simulink model "VCU_CS75_9_30"  (R2014a)
settings: Solver=FixedStepDiscrete  StartTime=0.0  StopTime=25  FixedStep=0.0005  RelTol=1e-3
undefined symbols (not defined in the file or in its folder): APAStatus_2D4, ecucoder_acal, I_SW01_L, LDW, ST_comd, TX2D4
libraries: simulink x881, ec5744lib x37
(part 24 of 30)

== system VCU_CS75_9_30/长安CS75底盘程序，20ms一次/BSW_Input/CAN1_Rx/BCM_3DF/ReceiveMessages/Subsystem/BCM_3DF1 ==
  input : Inport
  BCM_AmbientLightColorFeedback_Ad : Sum
  BCM_AmbientLightColorFeedback_Convert : DataTypeConversion  OutDataTypeStr=uint32
  BCM_AmbientLightColorFeedback_F : Gain
  BCM_AmbientLightColorFeedback_L : simulink/Logic and Bit Operations/Bitwise Operator  logicop=AND  UseBitMask=on  BitMask=255  BitMaskRealWorld=Stored Integer
  BCM_AmbientLightColorFeedback_O : Constant  Value=0  OutDataTypeStr=single
  BCM_AmbientLightColorFeedback_S : ArithShift
  BCM_AmbientLightColorFeedback_Sub : Subsystem
  BCM_AmbientLightColorFeedback_sat : Saturate  UpperLimit=255  LowerLimit=0
  BCM_AmbientLightColorFeedbackcv : DataTypeConversion
  BCM_CRC_Checksum_Ad : Sum
  BCM_CRC_Checksum_Convert : DataTypeConversion  OutDataTypeStr=uint32
  BCM_CRC_Checksum_F : Gain
  BCM_CRC_Checksum_L : simulink/Logic and Bit Operations/Bitwise Operator  logicop=AND  UseBitMask=on  BitMask=255  BitMaskRealWorld=Stored Integer
  BCM_CRC_Checksum_O : Constant  Value=0  OutDataTypeStr=single
  BCM_CRC_Checksum_S : ArithShift
  BCM_CRC_Checksum_Sub : Subsystem
  BCM_CRC_Checksum_sat : Saturate  UpperLimit=0  LowerLimit=0
  BCM_CRC_Checksumcv : DataTypeConversion
  BCM_DriveModeFeedback_Ad : Sum
  BCM_DriveModeFeedback_Convert : DataTypeConversion  OutDataTypeStr=uint32
  BCM_DriveModeFeedback_F : Gain
  BCM_DriveModeFeedback_L : simulink/Logic and Bit Operations/Bitwise Operator  logicop=AND  UseBitMask=on  BitMask=48  BitMaskRealWorld=Stored Integer
  BCM_DriveModeFeedback_O : Constant  Value=0  OutDataTypeStr=single
  BCM_DriveModeFeedback_S : ArithShift  BitShiftNumber=4
  BCM_DriveModeFeedback_Sub : Subsystem
  BCM_DriveModeFeedback_sat : Saturate  UpperLimit=3  LowerLimit=0
  BCM_DriveModeFeedbackcv : DataTypeConversion
  BCM_DriveModeStatus_Ad : Sum
  BCM_DriveModeStatus_Convert : DataTypeConversion  OutDataTypeStr=uint32
  BCM_DriveModeStatus_F : Gain
  BCM_DriveModeStatus_L : simulink/Logic and Bit Operations/Bitwise Operator  logicop=AND  UseBitMask=on  BitMask=15  BitMaskRealWorld=Stored Integer
  BCM_DriveModeStatus_O : Constant  Value=0  OutDataTypeStr=single
  BCM_DriveModeStatus_S : ArithShift
  BCM_DriveModeStatus_Sub : Subsystem
  BCM_DriveModeStatus_sat : Saturate  UpperLimit=15  LowerLimit=0
  BCM_DriveModeStatuscv : DataTypeConversion
  BCM_DriveMode_Ad : Sum
  BCM_DriveMode_Convert : DataTypeConversion  OutDataTypeStr=uint32
  BCM_DriveMode_F : Gain
  BCM_DriveMode_L : simulink/Logic and Bit Operations/Bitwise Operator  logicop=AND  UseBitMask=on  BitMask=240  BitMaskRealWorld=Stored Integer
  BCM_DriveMode_O : Constant  Value=0  OutDataTypeStr=single
  BCM_DriveMode_S : ArithShift  BitShiftNumber=4
  BCM_DriveMode_Sub : Subsystem
  BCM_DriveMode_sat : Saturate  UpperLimit=0  LowerLimit=0
  BCM_DriveModecv : DataTypeConversion
  BCM_EPSTorqueModeFeedback_Ad : Sum
  BCM_EPSTorqueModeFeedback_Convert : DataTypeConversion  OutDataTypeStr=uint32
  BCM_EPSTorqueModeFeedback_F : Gain
  BCM_EPSTorqueModeFeedback_L : simulink/Logic and Bit Operations/Bitwise Operator  logicop=AND  UseBitMask=on  BitMask=192  BitMaskRealWorld=Stored Integer
  BCM_EPSTorqueModeFeedback_O : Constant  Value=0  OutDataTypeStr=single
  BCM_EPSTorqueModeFeedback_S : ArithShift  BitShiftNumber=6
  BCM_EPSTorqueModeFeedback_Sub : Subsystem
  BCM_EPSTorqueModeFeedback_sat : Saturate  UpperLimit=3  LowerLimit=0
  BCM_EPSTorqueModeFeedbackcv : DataTypeConversion
  BCM_EPSTorqueMode_Ad : Sum
  BCM_EPSTorqueMode_Convert : DataTypeConversion  OutDataTypeStr=uint32
  BCM_EPSTorqueMode_F : Gain
  BCM_EPSTorqueMode_L : simulink/Logic and Bit Operations/Bitwise Operator  logicop=AND  UseBitMask=on  BitMask=6  BitMaskRealWorld=Stored Integer
  BCM_EPSTorqueMode_O : Constant  Value=0  OutDataTypeStr=single
  BCM_EPSTorqueMode_S : ArithShift  BitShiftNumber=1
  BCM_EPSTorqueMode_Sub : Subsystem
  BCM_EPSTorqueMode_sat : Saturate  UpperLimit=3  LowerLimit=0
  BCM_EPSTorqueModecv : DataTypeConversion
  BCM_RollingCounter_Ad : Sum
  BCM_RollingCounter_Convert : DataTypeConversion  OutDataTypeStr=uint32
  BCM_RollingCounter_F : Gain
  BCM_RollingCounter_L : simulink/Logic and Bit Operations/Bitwise Operator  logicop=AND  UseBitMask=on  BitMask=15  BitMaskRealWorld=Stored Integer
  BCM_RollingCounter_O : Constant  Value=0  OutDataTypeStr=single
  BCM_RollingCounter_S : ArithShift
  BCM_RollingCounter_Sub : Subsystem
  BCM_RollingCounter_sat : Saturate  UpperLimit=0  LowerLimit=0
  BCM_RollingCountercv : DataTypeConversion
  Demux : Demux  Outputs=8
  BCM_DriveMode_Out : Outport
  BCM_EPSTorqueMode_Out : Outport  Port=2
  BCM_DriveModeStatus_Out : Outport  Port=3
  BCM_DriveModeFeedback_Out : Outport  Port=4
  BCM_EPSTorqueModeFeedback_Out : Outport  Port=5
  BCM_AmbientLightColorFeedback_Out : Outport  Port=6
  BCM_RollingCounter_Out : Outport  Port=7
  BCM_CRC_Checksum_Out : Outport  Port=8
  wires:
  input/1 -> Demux/1
  BCM_CRC_Checksumcv/1 -> BCM_CRC_Checksum_F/1
  BCM_CRC_Checksum_S/1 -> BCM_CRC_Checksumcv/1
  BCM_CRC_Checksum_L/1 -> BCM_CRC_Checksum_S/1
  BCM_CRC_Checksum_Convert/1 -> BCM_CRC_Checksum_L/1
  BCM_CRC_Checksum_Sub/1(Out1) -> BCM_CRC_Checksum_Convert/1
  Demux/8 -> BCM_CRC_Checksum_Sub/1(In1)
  BCM_CRC_Checksum_sat/1 -> BCM_CRC_Checksum_Out/1
  BCM_CRC_Checksum_Ad/1 -> BCM_CRC_Checksum_sat/1
  BCM_CRC_Checksum_O/1 -> BCM_CRC_Checksum_Ad/2
  BCM_CRC_Checksum_F/1 -> BCM_CRC_Checksum_Ad/1
  BCM_RollingCountercv/1 -> BCM_RollingCounter_F/1
  BCM_RollingCounter_S/1 -> BCM_RollingCountercv/1
  BCM_RollingCounter_L/1 -> BCM_RollingCounter_S/1
  BCM_RollingCounter_Convert/1 -> BCM_RollingCounter_L/1
  BCM_RollingCounter_Sub/1(Out1) -> BCM_RollingCounter_Convert/1
  Demux/7 -> BCM_RollingCounter_Sub/1(In1)
  BCM_RollingCounter_sat/1 -> BCM_RollingCounter_Out/1
  BCM_RollingCounter_Ad/1 -> BCM_RollingCounter_sat/1
  BCM_RollingCounter_O/1 -> BCM_RollingCounter_Ad/2
  BCM_RollingCounter_F/1 -> BCM_RollingCounter_Ad/1
  BCM_AmbientLightColorFeedbackcv/1 -> BCM_AmbientLightColorFeedback_F/1
  BCM_AmbientLightColorFeedback_S/1 -> BCM_AmbientLightColorFeedbackcv/1
  BCM_AmbientLightColorFeedback_L/1 -> BCM_AmbientLightColorFeedback_S/1
  BCM_AmbientLightColorFeedback_Convert/1 -> BCM_AmbientLightColorFeedback_L/1
  BCM_AmbientLightColorFeedback_Sub/1(Out1) -> BCM_AmbientLightColorFeedback_Convert/1
  Demux/4 -> BCM_AmbientLightColorFeedback_Sub/1(In1)
  BCM_AmbientLightColorFeedback_sat/1 -> BCM_AmbientLightColorFeedback_Out/1
  BCM_AmbientLightColorFeedback_Ad/1 -> BCM_AmbientLightColorFeedback_sat/1
  BCM_AmbientLightColorFeedback_O/1 -> BCM_AmbientLightColorFeedback_Ad/2
  BCM_AmbientLightColorFeedback_F/1 -> BCM_AmbientLightColorFeedback_Ad/1
  BCM_EPSTorqueModeFeedbackcv/1 -> BCM_EPSTorqueModeFeedback_F/1
  BCM_EPSTorqueModeFeedback_S/1 -> BCM_EPSTorqueModeFeedbackcv/1
  BCM_EPSTorqueModeFeedback_L/1 -> BCM_EPSTorqueModeFeedback_S/1
  BCM_EPSTorqueModeFeedback_Convert/1 -> BCM_EPSTorqueModeFeedback_L/1
  BCM_EPSTorqueModeFeedback_Sub/1(Out1) -> BCM_EPSTorqueModeFeedback_Convert/1
  BCM_EPSTorqueModeFeedback_sat/1 -> BCM_EPSTorqueModeFeedback_Out/1
  BCM_EPSTorqueModeFeedback_Ad/1 -> BCM_EPSTorqueModeFeedback_sat/1
  BCM_EPSTorqueModeFeedback_O/1 -> BCM_EPSTorqueModeFeedback_Ad/2
  BCM_EPSTorqueModeFeedback_F/1 -> BCM_EPSTorqueModeFeedback_Ad/1
  BCM_DriveModeFeedbackcv/1 -> BCM_DriveModeFeedback_F/1
  BCM_DriveModeFeedback_S/1 -> BCM_DriveModeFeedbackcv/1
  BCM_DriveModeFeedback_L/1 -> BCM_DriveModeFeedback_S/1
  BCM_DriveModeFeedback_Convert/1 -> BCM_DriveModeFeedback_L/1
  BCM_DriveModeFeedback_Sub/1(Out1) -> BCM_DriveModeFeedback_Convert/1
  BCM_DriveModeFeedback_sat/1 -> BCM_DriveModeFeedback_Out/1
  BCM_DriveModeFeedback_Ad/1 -> BCM_DriveModeFeedback_sat/1
  BCM_DriveModeFeedback_O/1 -> BCM_DriveModeFeedback_Ad/2
  BCM_DriveModeFeedback_F/1 -> BCM_DriveModeFeedback_Ad/1
  BCM_DriveModeStatuscv/1 -> BCM_DriveModeStatus_F/1
  BCM_DriveModeStatus_S/1 -> BCM_DriveModeStatuscv/1
  BCM_DriveModeStatus_L/1 -> BCM_DriveModeStatus_S/1
  BCM_DriveModeStatus_Convert/1 -> BCM_DriveModeStatus_L/1
  BCM_DriveModeStatus_Sub/1(Out1) -> BCM_DriveModeStatus_Convert/1
  Demux/3 -> BCM_EPSTorqueModeFeedback_Sub/1(In1), BCM_DriveModeFeedback_Sub/1(In1), BCM_DriveModeStatus_Sub/1(In1)
  BCM_DriveModeStatus_sat/1 -> BCM_DriveModeStatus_Out/1
  BCM_DriveModeStatus_Ad/1 -> BCM_DriveModeStatus_sat/1
  BCM_DriveModeStatus_O/1 -> BCM_DriveModeStatus_Ad/2
  BCM_DriveModeStatus_F/1 -> BCM_DriveModeStatus_Ad/1
  BCM_EPSTorqueModecv/1 -> BCM_EPSTorqueMode_F/1
  BCM_EPSTorqueMode_S/1 -> BCM_EPSTorqueModecv/1
  BCM_EPSTorqueMode_L/1 -> BCM_EPSTorqueMode_S/1
  BCM_EPSTorqueMode_Convert/1 -> BCM_EPSTorqueMode_L/1
  BCM_EPSTorqueMode_Sub/1(Out1) -> BCM_EPSTorqueMode_Convert/1
  Demux/2 -> BCM_EPSTorqueMode_Sub/1(In1)
  BCM_EPSTorqueMode_sat/1 -> BCM_EPSTorqueMode_Out/1
  BCM_EPSTorqueMode_Ad/1 -> BCM_EPSTorqueMode_sat/1
  BCM_EPSTorqueMode_O/1 -> BCM_EPSTorqueMode_Ad/2
  BCM_EPSTorqueMode_F/1 -> BCM_EPSTorqueMode_Ad/1
  BCM_DriveModecv/1 -> BCM_DriveMode_F/1
  BCM_DriveMode_S/1 -> BCM_DriveModecv/1
  BCM_DriveMode_L/1 -> BCM_DriveMode_S/1
  BCM_DriveMode_Convert/1 -> BCM_DriveMode_L/1
  BCM_DriveMode_Sub/1(Out1) -> BCM_DriveMode_Convert/1
  Demux/1 -> BCM_DriveMode_Sub/1(In1)
  BCM_DriveMode_sat/1 -> BCM_DriveMode_Out/1
  BCM_DriveMode_Ad/1 -> BCM_DriveMode_sat/1
  BCM_DriveMode_O/1 -> BCM_DriveMode_Ad/2
  BCM_DriveMode_F/1 -> BCM_DriveMode_Ad/1

== system VCU_CS75_9_30/长安CS75底盘程序，20ms一次/BSW_Input/CAN1_Rx/EMS_205/ReceiveMessages/Subsystem/EMS ==
  input : Inport
  Demux : Demux  Outputs=8
  EMS_CheckSum_205_Ad : Sum
  EMS_CheckSum_205_Convert : DataTypeConversion  OutDataTypeStr=uint32
  EMS_CheckSum_205_F : Gain
  EMS_CheckSum_205_L : simulink/Logic and Bit Operations/Bitwise Operator  logicop=AND  UseBitMask=on  BitMask=240  BitMaskRealWorld=Stored Integer
  EMS_CheckSum_205_O : Constant  Value=0  OutDataTypeStr=single
  EMS_CheckSum_205_S : ArithShift  BitShiftNumber=4
  EMS_CheckSum_205_Sub : Subsystem
  EMS_CheckSum_205_sat : Saturate  UpperLimit=15  LowerLimit=0
  EMS_CheckSum_205cv : DataTypeConversion
  EMS_ESPTorqReuestAvailability_Ad : Sum
  EMS_ESPTorqReuestAvailability_Convert : DataTypeConversion  OutDataTypeStr=uint32
  EMS_ESPTorqReuestAvailability_F : Gain
  EMS_ESPTorqReuestAvailability_L : simulink/Logic and Bit Operations/Bitwise Operator  logicop=AND  UseBitMask=on  BitMask=2  BitMaskRealWorld=Stored Integer
  EMS_ESPTorqReuestAvailability_O : Constant  Value=0  OutDataTypeStr=single
  EMS_ESPTorqReuestAvailability_S : ArithShift  BitShiftNumber=1
  EMS_ESPTorqReuestAvailability_Sub : Subsystem
  EMS_ESPTorqReuestAvailability_sat : Saturate  UpperLimit=1  LowerLimit=0  OutDataTypeStr=Inherit: Inherit via back propagation
  EMS_ESPTorqReuestAvailabilitycv : DataTypeConversion
  EMS_FrictionalTorq_Ad : Sum
  EMS_FrictionalTorq_Convert : DataTypeConversion  OutDataTypeStr=uint32
  EMS_FrictionalTorq_F : Gain  Gain=0.001526
  EMS_FrictionalTorq_L : simulink/Logic and Bit Operations/Bitwise Operator  logicop=AND  UseBitMask=on  BitMask=65535  BitMaskRealWorld=Stored Integer
  EMS_FrictionalTorq_O : Constant  Value=0  OutDataTypeStr=single
  EMS_FrictionalTorq_S : ArithShift
  EMS_FrictionalTorq_Sub : Subsystem
  EMS_FrictionalTorq_sat : Saturate  UpperLimit=99.9988  LowerLimit=0
  EMS_FrictionalTorqcv : DataTypeConversion
  EMS_FrictionalTorqinput4_Ad : Sum
  EMS_FrictionalTorqinput4_C : Constant  Value=256
  EMS_FrictionalTorqinput4_P : Product
  EMS_IndicatedDriverReqTorq_Ad : Sum
  EMS_IndicatedDriverReqTorq_Convert : DataTypeConversion  OutDataTypeStr=uint32
  EMS_IndicatedDriverReqTorq_F : Gain  Gain=0.001526
  EMS_IndicatedDriverReqTorq_L : simulink/Logic and Bit Operations/Bitwise Operator  logicop=AND  UseBitMask=on  BitMask=65535  BitMaskRealWorld=Stored Integer
  EMS_IndicatedDriverReqTorq_O : Constant  Value=0  OutDataTypeStr=single
  EMS_IndicatedDriverReqTorq_S : ArithShift
  EMS_IndicatedDriverReqTorq_Sub : Subsystem
  EMS_IndicatedDriverReqTorq_sat : Saturate  UpperLimit=99.9988  LowerLimit=0
  EMS_IndicatedDriverReqTorqcv : DataTypeConversion
  EMS_IndicatedDriverReqTorqinput2_Ad : Sum
  EMS_IndicatedDriverReqTorqinput2_C : Constant  Value=256
  EMS_IndicatedDriverReqTorqinput2_P : Product
  EMS_IndicatedRealEngTorq_Ad : Sum
  EMS_IndicatedRealEngTorq_Convert : DataTypeConversion  OutDataTypeStr=uint32
  EMS_IndicatedRealEngTorq_F : Gain  Gain=0.001526
  EMS_IndicatedRealEngTorq_L : simulink/Logic and Bit Operations/Bitwise Operator  logicop=AND  UseBitMask=on  BitMask=65535  BitMaskRealWorld=Stored Integer
  EMS_IndicatedRealEngTorq_O : Constant  Value=0  OutDataTypeStr=single
  EMS_IndicatedRealEngTorq_S : ArithShift
  EMS_IndicatedRealEngTorq_Sub : Subsystem
  EMS_IndicatedRealEngTorq_sat : Saturate  UpperLimit=99.9988  LowerLimit=0
  EMS_IndicatedRealEngTorqcv : DataTypeConversion
  EMS_IndicatedRealEngTorqinput6_Ad : Sum
  EMS_IndicatedRealEngTorqinput6_C : Constant  Value=256
  EMS_IndicatedRealEngTorqinput6_P : Product
  EMS_RollingCounter_id205_Ad : Sum
  EMS_RollingCounter_id205_Convert : DataTypeConversion  OutDataTypeStr=uint32
  EMS_RollingCounter_id205_F : Gain
  EMS_RollingCounter_id205_L : simulink/Logic and Bit Operations/Bitwise Operator  logicop=AND  UseBitMask=on  BitMask=15  BitMaskRealWorld=Stored Integer
  EMS_RollingCounter_id205_O : Constant  Value=0  OutDataTypeStr=single
  EMS_RollingCounter_id205_S : ArithShift
  EMS_RollingCounter_id205_Sub : Subsystem
  EMS_RollingCounter_id205_sat : Saturate  UpperLimit=15  LowerLimit=0
  EMS_RollingCounter_id205cv : DataTypeConversion
  EMS_TorqFailure_Ad : Sum
  EMS_TorqFailure_Convert : DataTypeConversion  OutDataTypeStr=uint32
  EMS_TorqFailure_F : Gain
  EMS_TorqFailure_L : simulink/Logic and Bit Operations/Bitwise Operator  logicop=AND  UseBitMask=on  BitMask=128  BitMaskRealWorld=Stored Integer
  EMS_TorqFailure_O : Constant  Value=0  OutDataTypeStr=single
  EMS_TorqFailure_S : ArithShift  BitShiftNumber=7
  EMS_TorqFailure_Sub : Subsystem
  EMS_TorqFailure_sat : Saturate  UpperLimit=1  LowerLimit=0
  EMS_TorqFailurecv : DataTypeConversion
  EMS_ESPTorqReuestAvailability_Out : Outport
  EMS_TorqFailure_Out : Outport  Port=2
  EMS_IndicatedDriverReqTorq_Out : Outport  Port=3
  EMS_FrictionalTorq_Out : Outport  Port=4
  EMS_IndicatedRealEngTorq_Out : Outport  Port=5
  EMS_RollingCounter_id205_Out : Outport  Port=6
  EMS_CheckSum_205_Out : Outport  Port=7
  wires:
  EMS_ESPTorqReuestAvailability_F/1 -> EMS_ESPTorqReuestAvailability_Ad/1
  EMS_ESPTorqReuestAvailability_O/1 -> EMS_ESPTorqReuestAvailability_Ad/2
  EMS_ESPTorqReuestAvailability_sat/1 -> EMS_ESPTorqReuestAvailability_Out/1
  Demux/1 -> EMS_ESPTorqReuestAvailability_Sub/1(In1), EMS_TorqFailure_Sub/1(In1)
  EMS_ESPTorqReuestAvailability_Sub/1(Out1) -> EMS_ESPTorqReuestAvailability_Convert/1
  EMS_ESPTorqReuestAvailability_Convert/1 -> EMS_ESPTorqReuestAvailability_L/1
  EMS_ESPTorqReuestAvailability_L/1 -> EMS_ESPTorqReuestAvailability_S/1
  EMS_ESPTorqReuestAvailability_S/1 -> EMS_ESPTorqReuestAvailabilitycv/1
  EMS_ESPTorqReuestAvailabilitycv/1 -> EMS_ESPTorqReuestAvailability_F/1
  EMS_TorqFailure_F/1 -> EMS_TorqFailure_Ad/1
  EMS_TorqFailure_O/1 -> EMS_TorqFailure_Ad/2
  EMS_TorqFailure_Ad/1 -> EMS_TorqFailure_sat/1
  EMS_TorqFailure_sat/1 -> EMS_TorqFailure_Out/1
  EMS_TorqFailure_Sub/1(Out1) -> EMS_TorqFailure_Convert/1
  EMS_TorqFailure_Convert/1 -> EMS_TorqFailure_L/1
  EMS_TorqFailure_L/1 -> EMS_TorqFailure_S/1
  EMS_TorqFailure_S/1 -> EMS_TorqFailurecv/1
  EMS_TorqFailurecv/1 -> EMS_TorqFailure_F/1
  EMS_IndicatedDriverReqTorq_F/1 -> EMS_IndicatedDriverReqTorq_Ad/1
  EMS_IndicatedDriverReqTorq_O/1 -> EMS_IndicatedDriverReqTorq_Ad/2
  EMS_IndicatedDriverReqTorq_Ad/1 -> EMS_IndicatedDriverReqTorq_sat/1
  EMS_IndicatedDriverReqTorq_sat/1 -> EMS_IndicatedDriverReqTorq_Out/1
  Demux/2 -> EMS_IndicatedDriverReqTorqinput2_P/1
  EMS_IndicatedDriverReqTorqinput2_C/1 -> EMS_IndicatedDriverReqTorqinput2_P/2
  EMS_IndicatedDriverReqTorqinput2_P/1 -> EMS_IndicatedDriverReqTorqinput2_Ad/1
  Demux/3 -> EMS_IndicatedDriverReqTorqinput2_Ad/2
  EMS_IndicatedDriverReqTorqinput2_Ad/1 -> EMS_IndicatedDriverReqTorq_Sub/1(In1)
  EMS_IndicatedDriverReqTorq_Sub/1(Out1) -> EMS_IndicatedDriverReqTorq_Convert/1
  EMS_IndicatedDriverReqTorq_Convert/1 -> EMS_IndicatedDriverReqTorq_L/1
  EMS_IndicatedDriverReqTorq_L/1 -> EMS_IndicatedDriverReqTorq_S/1
  EMS_IndicatedDriverReqTorq_S/1 -> EMS_IndicatedDriverReqTorqcv/1
  EMS_IndicatedDriverReqTorqcv/1 -> EMS_IndicatedDriverReqTorq_F/1
  EMS_FrictionalTorq_F/1 -> EMS_FrictionalTorq_Ad/1
  EMS_FrictionalTorq_O/1 -> EMS_FrictionalTorq_Ad/2
  EMS_FrictionalTorq_Ad/1 -> EMS_FrictionalTorq_sat/1
  EMS_FrictionalTorq_sat/1 -> EMS_FrictionalTorq_Out/1
  Demux/4 -> EMS_FrictionalTorqinput4_P/1
  EMS_FrictionalTorqinput4_C/1 -> EMS_FrictionalTorqinput4_P/2
  EMS_FrictionalTorqinput4_P/1 -> EMS_FrictionalTorqinput4_Ad/1
  Demux/5 -> EMS_FrictionalTorqinput4_Ad/2
  EMS_FrictionalTorqinput4_Ad/1 -> EMS_FrictionalTorq_Sub/1(In1)
  EMS_FrictionalTorq_Sub/1(Out1) -> EMS_FrictionalTorq_Convert/1
  EMS_FrictionalTorq_Convert/1 -> EMS_FrictionalTorq_L/1
  EMS_FrictionalTorq_L/1 -> EMS_FrictionalTorq_S/1
  EMS_FrictionalTorq_S/1 -> EMS_FrictionalTorqcv/1
  EMS_FrictionalTorqcv/1 -> EMS_FrictionalTorq_F/1
  EMS_IndicatedRealEngTorq_F/1 -> EMS_IndicatedRealEngTorq_Ad/1
  EMS_IndicatedRealEngTorq_O/1 -> EMS_IndicatedRealEngTorq_Ad/2
  EMS_IndicatedRealEngTorq_Ad/1 -> EMS_IndicatedRealEngTorq_sat/1
  EMS_IndicatedRealEngTorq_sat/1 -> EMS_IndicatedRealEngTorq_Out/1
  Demux/6 -> EMS_IndicatedRealEngTorqinput6_P/1
  EMS_IndicatedRealEngTorqinput6_C/1 -> EMS_IndicatedRealEngTorqinput6_P/2
  EMS_IndicatedRealEngTorqinput6_P/1 -> EMS_IndicatedRealEngTorqinput6_Ad/1
  Demux/7 -> EMS_IndicatedRealEngTorqinput6_Ad/2
  EMS_IndicatedRealEngTorqinput6_Ad/1 -> EMS_IndicatedRealEngTorq_Sub/1(In1)
  EMS_IndicatedRealEngTorq_Sub/1(Out1) -> EMS_IndicatedRealEngTorq_Convert/1
  EMS_IndicatedRealEngTorq_Convert/1 -> EMS_IndicatedRealEngTorq_L/1
  EMS_IndicatedRealEngTorq_L/1 -> EMS_IndicatedRealEngTorq_S/1
  EMS_IndicatedRealEngTorq_S/1 -> EMS_IndicatedRealEngTorqcv/1
  EMS_IndicatedRealEngTorqcv/1 -> EMS_IndicatedRealEngTorq_F/1
  EMS_RollingCounter_id205_F/1 -> EMS_RollingCounter_id205_Ad/1
  EMS_RollingCounter_id205_O/1 -> EMS_RollingCounter_id205_Ad/2
  EMS_RollingCounter_id205_Ad/1 -> EMS_RollingCounter_id205_sat/1
  EMS_RollingCounter_id205_sat/1 -> EMS_RollingCounter_id205_Out/1
  Demux/8 -> EMS_RollingCounter_id205_Sub/1(In1), EMS_CheckSum_205_Sub/1(In1)
  EMS_RollingCounter_id205_Sub/1(Out1) -> EMS_RollingCounter_id205_Convert/1
  EMS_RollingCounter_id205_Convert/1 -> EMS_RollingCounter_id205_L/1
  EMS_RollingCounter_id205_L/1 -> EMS_RollingCounter_id205_S/1
  EMS_RollingCounter_id205_S/1 -> EMS_RollingCounter_id205cv/1
  EMS_RollingCounter_id205cv/1 -> EMS_RollingCounter_id205_F/1
  EMS_CheckSum_205_F/1 -> EMS_CheckSum_205_Ad/1
  EMS_CheckSum_205_O/1 -> EMS_CheckSum_205_Ad/2
  EMS_CheckSum_205_Ad/1 -> EMS_CheckSum_205_sat/1
  EMS_CheckSum_205_sat/1 -> EMS_CheckSum_205_Out/1
  EMS_CheckSum_205_Sub/1(Out1) -> EMS_CheckSum_205_Convert/1
  EMS_CheckSum_205_Convert/1 -> EMS_CheckSum_205_L/1
  EMS_CheckSum_205_L/1 -> EMS_CheckSum_205_S/1
  EMS_CheckSum_205_S/1 -> EMS_CheckSum_205cv/1
  EMS_CheckSum_205cv/1 -> EMS_CheckSum_205_F/1
  input/1 -> Demux/1
  EMS_ESPTorqReuestAvailability_Ad/1 -> EMS_ESPTorqReuestAvailability_sat/1

== system VCU_CS75_9_30/长安CS75底盘程序，20ms一次/BSW_Input/CAN1_Rx/EMS_255/ReceiveMessages/Subsystem/EMS ==
  input : Inport
  Demux : Demux  Outputs=8
  EMS_AccPedal_Ad : Sum
  EMS_AccPedal_Convert : DataTypeConversion  OutDataTypeStr=uint32
  EMS_AccPedal_F : Gain  Gain=0.392
  EMS_AccPedal_L : simulink/Logic and Bit Operations/Bitwise Operator  logicop=AND  UseBitMask=on  BitMask=255  BitMaskRealWorld=Stored Integer
  EMS_AccPedal_O : Constant  Value=0  OutDataTypeStr=single
  EMS_AccPedal_S : ArithShift
  EMS_AccPedal_Sub : Subsystem
  EMS_AccPedal_sat : Saturate  UpperLimit=99.568  LowerLimit=0
  EMS_AccPedalcv : DataTypeConversion
  EMS_AccpedelError_Ad : Sum
  EMS_AccpedelError_Convert : DataTypeConversion  OutDataTypeStr=uint32
  EMS_AccpedelError_F : Gain
  EMS_AccpedelError_L : simulink/Logic and Bit Operations/Bitwise Operator  logicop=AND  UseBitMask=on  BitMask=4  BitMaskRealWorld=Stored Integer
  EMS_AccpedelError_O : Constant  Value=0  OutDataTypeStr=single
  EMS_AccpedelError_S : ArithShift  BitShiftNumber=2
  EMS_AccpedelError_Sub : Subsystem
  EMS_AccpedelError_sat : Saturate  UpperLimit=1  LowerLimit=0
  EMS_AccpedelErrorcv : DataTypeConversion
  EMS_BrakePedalStatus_Ad : Sum
  EMS_BrakePedalStatus_Convert : DataTypeConversion  OutDataTypeStr=uint32
  EMS_BrakePedalStatus_F : Gain
  EMS_BrakePedalStatus_L : simulink/Logic and Bit Operations/Bitwise Operator  logicop=AND  UseBitMask=on  BitMask=192  BitMaskRealWorld=Stored Integer
  EMS_BrakePedalStatus_O : Constant  Value=0  OutDataTypeStr=single
  EMS_BrakePedalStatus_S : ArithShift  BitShiftNumber=6
  EMS_BrakePedalStatus_Sub : Subsystem
  EMS_BrakePedalStatus_sat : Saturate  UpperLimit=3  LowerLimit=0
  EMS_BrakePedalStatuscv : DataTypeConversion
  EMS_CheckSum_255_Ad : Sum
  EMS_CheckSum_255_Convert : DataTypeConversion  OutDataTypeStr=uint32
  EMS_CheckSum_255_F : Gain
  EMS_CheckSum_255_L : simulink/Logic and Bit Operations/Bitwise Operator  logicop=AND  UseBitMask=on  BitMask=240  BitMaskRealWorld=Stored Integer
  EMS_CheckSum_255_O : Constant  Value=0  OutDataTypeStr=single
  EMS_CheckSum_255_S : ArithShift  BitShiftNumber=4
  EMS_CheckSum_255_Sub : Subsystem
  EMS_CheckSum_255_sat : Saturate  UpperLimit=15  LowerLimit=0
  EMS_CheckSum_255cv : DataTypeConversion
  EMS_EngineSpeedError_Ad : Sum
  EMS_EngineSpeedError_Convert : DataTypeConversion  OutDataTypeStr=uint32
  EMS_EngineSpeedError_F : Gain
  EMS_EngineSpeedError_L : simulink/Logic and Bit Operations/Bitwise Operator  logicop=AND  UseBitMask=on  BitMask=16  BitMaskRealWorld=Stored Integer
  EMS_EngineSpeedError_O : Constant  Value=0  OutDataTypeStr=single
  EMS_EngineSpeedError_S : ArithShift  BitShiftNumber=4
  EMS_EngineSpeedError_Sub : Subsystem
  EMS_EngineSpeedError_sat : Saturate  UpperLimit=1  LowerLimit=0
  EMS_EngineSpeedErrorcv : DataTypeConversion
  EMS_EngineSpeed_Ad : Sum
  EMS_EngineSpeed_Convert : DataTypeConversion  OutDataTypeStr=uint32
  EMS_EngineSpeed_F : Gain  Gain=0.25
  EMS_EngineSpeed_L : simulink/Logic and Bit Operations/Bitwise Operator  logicop=AND  UseBitMask=on  BitMask=65535  BitMaskRealWorld=Stored Integer
  EMS_EngineSpeed_O : Constant  Value=0  OutDataTypeStr=single
  EMS_EngineSpeed_S : ArithShift
  EMS_EngineSpeed_Sub : Subsystem
  EMS_EngineSpeed_sat : Saturate  UpperLimit=16383.5  LowerLimit=0
  EMS_EngineSpeedcv : DataTypeConversion
  EMS_EngineSpeedinput3_Ad : Sum
  EMS_EngineSpeedinput3_C : Constant  Value=256
  EMS_EngineSpeedinput3_P : Product
  EMS_RollingCounter_id255_Ad : Sum
  EMS_RollingCounter_id255_Convert : DataTypeConversion  OutDataTypeStr=uint32
  EMS_RollingCounter_id255_F : Gain
  EMS_RollingCounter_id255_L : simulink/Logic and Bit Operations/Bitwise Operator  logicop=AND  UseBitMask=on  BitMask=15  BitMaskRealWorld=Stored Integer
  EMS_RollingCounter_id255_O : Constant  Value=0  OutDataTypeStr=single
  EMS_RollingCounter_id255_S : ArithShift
  EMS_RollingCounter_id255_Sub : Subsystem
  EMS_RollingCounter_id255_sat : Saturate  UpperLimit=15  LowerLimit=0
  EMS_RollingCounter_id255cv : DataTypeConversion
  EMS_BrakePedalStatus_Out : Outport
  EMS_AccpedelError_Out : Outport  Port=2
  EMS_EngineSpeedError_Out : Outport  Port=3
  EMS_EngineSpeed_Out : Outport  Port=4
  EMS_AccPedal_Out : Outport  Port=5
  EMS_RollingCounter_id255_Out : Outport  Port=6
  EMS_CheckSum_255_Out : Outport  Port=7
  wires:
  EMS_BrakePedalStatus_F/1 -> EMS_BrakePedalStatus_Ad/1
  EMS_BrakePedalStatus_O/1 -> EMS_BrakePedalStatus_Ad/2
  EMS_BrakePedalStatus_Ad/1 -> EMS_BrakePedalStatus_sat/1
  EMS_BrakePedalStatus_sat/1 -> EMS_BrakePedalStatus_Out/1
  Demux/1 -> EMS_BrakePedalStatus_Sub/1(In1)
  EMS_BrakePedalStatus_Sub/1(Out1) -> EMS_BrakePedalStatus_Convert/1
  EMS_BrakePedalStatus_Convert/1 -> EMS_BrakePedalStatus_L/1
  EMS_BrakePedalStatus_L/1 -> EMS_BrakePedalStatus_S/1
  EMS_BrakePedalStatus_S/1 -> EMS_BrakePedalStatuscv/1
  EMS_BrakePedalStatuscv/1 -> EMS_BrakePedalStatus_F/1
  EMS_AccpedelError_F/1 -> EMS_AccpedelError_Ad/1
  EMS_AccpedelError_O/1 -> EMS_AccpedelError_Ad/2
  EMS_AccpedelError_Ad/1 -> EMS_AccpedelError_sat/1
  EMS_AccpedelError_sat/1 -> EMS_AccpedelError_Out/1
  Demux/2 -> EMS_AccpedelError_Sub/1(In1), EMS_EngineSpeedError_Sub/1(In1)
  EMS_AccpedelError_Sub/1(Out1) -> EMS_AccpedelError_Convert/1
  EMS_AccpedelError_Convert/1 -> EMS_AccpedelError_L/1
  EMS_AccpedelError_L/1 -> EMS_AccpedelError_S/1
  EMS_AccpedelError_S/1 -> EMS_AccpedelErrorcv/1
  EMS_AccpedelErrorcv/1 -> EMS_AccpedelError_F/1
  EMS_EngineSpeedError_F/1 -> EMS_EngineSpeedError_Ad/1
  EMS_EngineSpeedError_O/1 -> EMS_EngineSpeedError_Ad/2
  EMS_EngineSpeedError_Ad/1 -> EMS_EngineSpeedError_sat/1
  EMS_EngineSpeedError_sat/1 -> EMS_EngineSpeedError_Out/1
  EMS_EngineSpeedError_Sub/1(Out1) -> EMS_EngineSpeedError_Convert/1
  EMS_EngineSpeedError_Convert/1 -> EMS_EngineSpeedError_L/1
  EMS_EngineSpeedError_L/1 -> EMS_EngineSpeedError_S/1
  EMS_EngineSpeedError_S/1 -> EMS_EngineSpeedErrorcv/1
  EMS_EngineSpeedErrorcv/1 -> EMS_EngineSpeedError_F/1
  EMS_EngineSpeed_F/1 -> EMS_EngineSpeed_Ad/1
  EMS_EngineSpeed_O/1 -> EMS_EngineSpeed_Ad/2
  EMS_EngineSpeed_Ad/1 -> EMS_EngineSpeed_sat/1
  EMS_EngineSpeed_sat/1 -> EMS_EngineSpeed_Out/1
  Demux/3 -> EMS_EngineSpeedinput3_P/1
  EMS_EngineSpeedinput3_C/1 -> EMS_EngineSpeedinput3_P/2
  EMS_EngineSpeedinput3_P/1 -> EMS_EngineSpeedinput3_Ad/1
  Demux/4 -> EMS_EngineSpeedinput3_Ad/2
  EMS_EngineSpeedinput3_Ad/1 -> EMS_EngineSpeed_Sub/1(In1)
  EMS_EngineSpeed_Sub/1(Out1) -> EMS_EngineSpeed_Convert/1
  EMS_EngineSpeed_Convert/1 -> EMS_EngineSpeed_L/1
  EMS_EngineSpeed_L/1 -> EMS_EngineSpeed_S/1
  EMS_EngineSpeed_S/1 -> EMS_EngineSpeedcv/1
  EMS_EngineSpeedcv/1 -> EMS_EngineSpeed_F/1
  EMS_AccPedal_F/1 -> EMS_AccPedal_Ad/1
  EMS_AccPedal_O/1 -> EMS_AccPedal_Ad/2
  EMS_AccPedal_Ad/1 -> EMS_AccPedal_sat/1
  EMS_AccPedal_sat/1 -> EMS_AccPedal_Out/1
  Demux/6 -> EMS_AccPedal_Sub/1(In1)
  EMS_AccPedal_Sub/1(Out1) -> EMS_AccPedal_Convert/1
  EMS_AccPedal_Convert/1 -> EMS_AccPedal_L/1
  EMS_AccPedal_L/1 -> EMS_AccPedal_S/1
  EMS_AccPedal_S/1 -> EMS_AccPedalcv/1
  EMS_AccPedalcv/1 -> EMS_AccPedal_F/1
  EMS_RollingCounter_id255_F/1 -> EMS_RollingCounter_id255_Ad/1
  EMS_RollingCounter_id255_O/1 -> EMS_RollingCounter_id255_Ad/2
  EMS_RollingCounter_id255_Ad/1 -> EMS_RollingCounter_id255_sat/1
  EMS_RollingCounter_id255_sat/1 -> EMS_RollingCounter_id255_Out/1
  Demux/8 -> EMS_RollingCounter_id255_Sub/1(In1), EMS_CheckSum_255_Sub/1(In1)
  EMS_RollingCounter_id255_Sub/1(Out1) -> EMS_RollingCounter_id255_Convert/1
  EMS_RollingCounter_id255_Convert/1 -> EMS_RollingCounter_id255_L/1
  EMS_RollingCounter_id255_L/1 -> EMS_RollingCounter_id255_S/1
  EMS_RollingCounter_id255_S/1 -> EMS_RollingCounter_id255cv/1
  EMS_RollingCounter_id255cv/1 -> EMS_RollingCounter_id255_F/1
  EMS_CheckSum_255_F/1 -> EMS_CheckSum_255_Ad/1
  EMS_CheckSum_255_O/1 -> EMS_CheckSum_255_Ad/2
  EMS_CheckSum_255_Ad/1 -> EMS_CheckSum_255_sat/1
  EMS_CheckSum_255_sat/1 -> EMS_CheckSum_255_Out/1
  EMS_CheckSum_255_Sub/1(Out1) -> EMS_CheckSum_255_Convert/1
  EMS_CheckSum_255_Convert/1 -> EMS_CheckSum_255_L/1
  EMS_CheckSum_255_L/1 -> EMS_CheckSum_255_S/1
  EMS_CheckSum_255_S/1 -> EMS_CheckSum_255cv/1
  EMS_CheckSum_255cv/1 -> EMS_CheckSum_255_F/1
  input/1 -> Demux/1

== system VCU_CS75_9_30/长安CS75底盘程序，20ms一次/BSW_Input/CAN1_Rx/EMS_265/ReceiveMessages/Subsystem/EMS_265xx ==
  input : Inport
  Demux : Demux  Outputs=8
  EMS_EngineStatus_Ad : Sum
  EMS_EngineStatus_Convert : DataTypeConversion  OutDataTypeStr=uint32
  EMS_EngineStatus_F : Gain
  EMS_EngineStatus_L : simulink/Logic and Bit Operations/Bitwise Operator  logicop=AND  UseBitMask=on  BitMask=192  BitMaskRealWorld=Stored Integer
  EMS_EngineStatus_O : Constant  Value=0  OutDataTypeStr=single
  EMS_EngineStatus_S : ArithShift  BitShiftNumber=6
  EMS_EngineStatus_Sub : Subsystem
  EMS_EngineStatus_sat : Saturate  UpperLimit=3  LowerLimit=0
  EMS_EngineStatuscv : DataTypeConversion
  EMS_FullLoadIndicatedTorq_Ad : Sum
  EMS_FullLoadIndicatedTorq_Convert : DataTypeConversion  OutDataTypeStr=uint32
  EMS_FullLoadIndicatedTorq_F : Gain  Gain=0.392
  EMS_FullLoadIndicatedTorq_L : simulink/Logic and Bit Operations/Bitwise Operator  logicop=AND  UseBitMask=on  BitMask=255  BitMaskRealWorld=Stored Integer
  EMS_FullLoadIndicatedTorq_O : Constant  Value=0  OutDataTypeStr=single
  EMS_FullLoadIndicatedTorq_S : ArithShift
  EMS_FullLoadIndicatedTorq_Sub : Subsystem
  EMS_FullLoadIndicatedTorq_sat : Saturate  UpperLimit=99.96  LowerLimit=0
  EMS_FullLoadIndicatedTorqcv : DataTypeConversion
  EMS_RollingCounter_id265_Ad : Sum
  EMS_RollingCounter_id265_Convert : DataTypeConversion  OutDataTypeStr=uint32
  EMS_RollingCounter_id265_F : Gain
  EMS_RollingCounter_id265_L : simulink/Logic and Bit Operations/Bitwise Operator  logicop=AND  UseBitMask=on  BitMask=15  BitMaskRealWorld=Stored Integer
  EMS_RollingCounter_id265_O : Constant  Value=0  OutDataTypeStr=single
  EMS_RollingCounter_id265_S : ArithShift
  EMS_RollingCounter_id265_Sub : Subsystem
  EMS_RollingCounter_id265_sat : Saturate  UpperLimit=15  LowerLimit=0
  EMS_RollingCounter_id265cv : DataTypeConversion
  EMS_TorqueConstant_Ad : Sum
  EMS_TorqueConstant_Convert : DataTypeConversion  OutDataTypeStr=uint32
  EMS_TorqueConstant_F : Gain  Gain=10
  EMS_TorqueConstant_L : simulink/Logic and Bit Operations/Bitwise Operator  logicop=AND  UseBitMask=on  BitMask=255  BitMaskRealWorld=Stored Integer
  EMS_TorqueConstant_O : Constant  Value=0  OutDataTypeStr=single
  EMS_TorqueConstant_S : ArithShift
  EMS_TorqueConstant_Sub : Subsystem
  EMS_TorqueConstant_sat : Saturate  UpperLimit=2540  LowerLimit=0
  EMS_TorqueConstantcv : DataTypeConversion
  EMS_FullLoadIndicatedTorq_Out : Outport
  EMS_TorqueConstant_Out : Outport  Port=2
  EMS_RollingCounter_id265_Out : Outport  Port=3
  EMS_EngineStatus_Out : Outport  Port=4
  wires:
  EMS_FullLoadIndicatedTorq_F/1 -> EMS_FullLoadIndicatedTorq_Ad/1
  EMS_FullLoadIndicatedTorq_O/1 -> EMS_FullLoadIndicatedTorq_Ad/2
  EMS_FullLoadIndicatedTorq_Ad/1 -> EMS_FullLoadIndicatedTorq_sat/1
  EMS_FullLoadIndicatedTorq_sat/1 -> EMS_FullLoadIndicatedTorq_Out/1
  Demux/3 -> EMS_FullLoadIndicatedTorq_Sub/1(In1)
  EMS_FullLoadIndicatedTorq_Sub/1(Out1) -> EMS_FullLoadIndicatedTorq_Convert/1
  EMS_FullLoadIndicatedTorq_Convert/1 -> EMS_FullLoadIndicatedTorq_L/1
  EMS_FullLoadIndicatedTorq_L/1 -> EMS_FullLoadIndicatedTorq_S/1
  EMS_FullLoadIndicatedTorq_S/1 -> EMS_FullLoadIndicatedTorqcv/1
  EMS_FullLoadIndicatedTorqcv/1 -> EMS_FullLoadIndicatedTorq_F/1
  EMS_TorqueConstant_F/1 -> EMS_TorqueConstant_Ad/1
  EMS_TorqueConstant_O/1 -> EMS_TorqueConstant_Ad/2
  EMS_TorqueConstant_Ad/1 -> EMS_TorqueConstant_sat/1
  EMS_TorqueConstant_sat/1 -> EMS_TorqueConstant_Out/1
  Demux/7 -> EMS_TorqueConstant_Sub/1(In1)
  EMS_TorqueConstant_Sub/1(Out1) -> EMS_TorqueConstant_Convert/1
  EMS_TorqueConstant_Convert/1 -> EMS_TorqueConstant_L/1
  EMS_TorqueConstant_L/1 -> EMS_TorqueConstant_S/1
  EMS_TorqueConstant_S/1 -> EMS_TorqueConstantcv/1
  EMS_TorqueConstantcv/1 -> EMS_TorqueConstant_F/1
  EMS_RollingCounter_id265_F/1 -> EMS_RollingCounter_id265_Ad/1
  EMS_RollingCounter_id265_O/1 -> EMS_RollingCounter_id265_Ad/2
  EMS_RollingCounter_id265_Ad/1 -> EMS_RollingCounter_id265_sat/1
  EMS_RollingCounter_id265_sat/1 -> EMS_RollingCounter_id265_Out/1
  Demux/8 -> EMS_RollingCounter_id265_Sub/1(In1), EMS_EngineStatus_Sub/1(In1)
  EMS_RollingCounter_id265_Sub/1(Out1) -> EMS_RollingCounter_id265_Convert/1
  EMS_RollingCounter_id265_Convert/1 -> EMS_RollingCounter_id265_L/1
  EMS_RollingCounter_id265_L/1 -> EMS_RollingCounter_id265_S/1
  EMS_RollingCounter_id265_S/1 -> EMS_RollingCounter_id265cv/1
  EMS_RollingCounter_id265cv/1 -> EMS_RollingCounter_id265_F/1
  EMS_EngineStatus_F/1 -> EMS_EngineStatus_Ad/1
  EMS_EngineStatus_O/1 -> EMS_EngineStatus_Ad/2
  EMS_EngineStatus_Ad/1 -> EMS_EngineStatus_sat/1
  EMS_EngineStatus_sat/1 -> EMS_EngineStatus_Out/1
  EMS_EngineStatus_Sub/1(Out1) -> EMS_EngineStatus_Convert/1
  EMS_EngineStatus_Convert/1 -> EMS_EngineStatus_L/1
  EMS_EngineStatus_L/1 -> EMS_EngineStatus_S/1
  EMS_EngineStatus_S/1 -> EMS_EngineStatuscv/1
  EMS_EngineStatuscv/1 -> EMS_EngineStatus_F/1
  input/1 -> Demux/1

== system VCU_CS75_9_30/长安CS75底盘程序，20ms一次/BSW_Input/CAN1_Rx/EMS_276/ReceiveMessages/Subsystem/EMS_2 ==
  input : Inport
  Demux : Demux  Outputs=8
  EMS_RealAccPedal_Ad : Sum
  EMS_RealAccPedal_Convert : DataTypeConversion  OutDataTypeStr=uint32
  EMS_RealAccPedal_F : Gain  Gain=0.392
  EMS_RealAccPedal_L : simulink/Logic and Bit Operations/Bitwise Operator  logicop=AND  UseBitMask=on  BitMask=255  BitMaskRealWorld=Stored Integer
  EMS_RealAccPedal_O : Constant  Value=0  OutDataTypeStr=single
  EMS_RealAccPedal_S : ArithShift
  EMS_RealAccPedal_Sub : Subsystem
  EMS_RealAccPedal_sat : Saturate  UpperLimit=99.96  LowerLimit=0
  EMS_RealAccPedalcv : DataTypeConversion
  EMS_RealAccPedal_Out : Outport
  wires:
  input/1 -> Demux/1
  EMS_RealAccPedalcv/1 -> EMS_RealAccPedal_F/1
  EMS_RealAccPedal_S/1 -> EMS_RealAccPedalcv/1
  EMS_RealAccPedal_L/1 -> EMS_RealAccPedal_S/1
  EMS_RealAccPedal_Convert/1 -> EMS_RealAccPedal_L/1
  EMS_RealAccPedal_Sub/1(Out1) -> EMS_RealAccPedal_Convert/1
  Demux/3 -> EMS_RealAccPedal_Sub/1(In1)
  EMS_RealAccPedal_sat/1 -> EMS_RealAccPedal_Out/1
  EMS_RealAccPedal_Ad/1 -> EMS_RealAccPedal_sat/1
  EMS_RealAccPedal_O/1 -> EMS_RealAccPedal_Ad/2
  EMS_RealAccPedal_F/1 -> EMS_RealAccPedal_Ad/1

== system VCU_CS75_9_30/长安CS75底盘程序，20ms一次/BSW_Input/CAN1_Rx/EPB_256/ReceiveMessages/Subsystem/EPB ==
  input : Inport
  Demux : Demux  Outputs=8
  EPB_Checksum_Ad : Sum
  EPB_Checksum_Convert : DataTypeConversion  OutDataTypeStr=uint32
  EPB_Checksum_F : Gain
  EPB_Checksum_L : simulink/Logic and Bit Operations/Bitwise Operator  logicop=AND  UseBitMask=on  BitMask=255  BitMaskRealWorld=Stored Integer
  EPB_Checksum_O : Constant  Value=0  OutDataTypeStr=single
  EPB_Checksum_S : ArithShift
  EPB_Checksum_Sub : Subsystem
  EPB_Checksum_sat : Saturate  UpperLimit=255  LowerLimit=0
  EPB_Checksumcv : DataTypeConversion
  EPB_FailStatus_Ad : Sum
  EPB_FailStatus_Convert : DataTypeConversion  OutDataTypeStr=uint32
  EPB_FailStatus_F : Gain
  EPB_FailStatus_L : simulink/Logic and Bit Operations/Bitwise Operator  logicop=AND  UseBitMask=on  BitMask=192  BitMaskRealWorld=Stored Integer
  EPB_FailStatus_O : Constant  Value=0  OutDataTypeStr=single
  EPB_FailStatus_S : ArithShift  BitShiftNumber=6
  EPB_FailStatus_Sub : Subsystem
  EPB_FailStatus_sat : Saturate  UpperLimit=3  LowerLimit=0
  EPB_FailStatuscv : DataTypeConversion
  EPB_FailureLamp_Ad : Sum
  EPB_FailureLamp_Convert : DataTypeConversion  OutDataTypeStr=uint32
  EPB_FailureLamp_F : Gain
  EPB_FailureLamp_L : simulink/Logic and Bit Operations/Bitwise Operator  logicop=AND  UseBitMask=on  BitMask=48  BitMaskRealWorld=Stored Integer
  EPB_FailureLamp_O : Constant  Value=0  OutDataTypeStr=single
  EPB_FailureLamp_S : ArithShift  BitShiftNumber=4
  EPB_FailureLamp_Sub : Subsystem
  EPB_FailureLamp_sat : Saturate  UpperLimit=3  LowerLimit=0
  EPB_FailureLampcv : DataTypeConversion
  EPB_FunctionLamp_Ad : Sum
  EPB_FunctionLamp_Convert : DataTypeConversion  OutDataTypeStr=uint32
  EPB_FunctionLamp_F : Gain
  EPB_FunctionLamp_L : simulink/Logic and Bit Operations/Bitwise Operator  logicop=AND  UseBitMask=on  BitMask=12  BitMaskRealWorld=Stored Integer
  EPB_FunctionLamp_O : Constant  Value=0  OutDataTypeStr=single
  EPB_FunctionLamp_S : ArithShift  BitShiftNumber=2
  EPB_FunctionLamp_Sub : Subsystem
  EPB_FunctionLamp_sat : Saturate  UpperLimit=3  LowerLimit=0
  EPB_FunctionLampcv : DataTypeConversion
  EPB_RollingCounter_id256_Ad : Sum
  EPB_RollingCounter_id256_Convert : DataTypeConversion  OutDataTypeStr=uint32
  EPB_RollingCounter_id256_F : Gain
  EPB_RollingCounter_id256_L : simulink/Logic and Bit Operations/Bitwise Operator  logicop=AND  UseBitMask=on  BitMask=15  BitMaskRealWorld=Stored Integer
  EPB_RollingCounter_id256_O : Constant  Value=0  OutDataTypeStr=single
  EPB_RollingCounter_id256_S : ArithShift
  EPB_RollingCounter_id256_Sub : Subsystem
  EPB_RollingCounter_id256_sat : Saturate  UpperLimit=15  LowerLimit=0
  EPB_RollingCounter_id256cv : DataTypeConversion
  EPB_Status_Ad : Sum
  EPB_Status_Convert : DataTypeConversion  OutDataTypeStr=uint32
  EPB_Status_F : Gain
  EPB_Status_L : simulink/Logic and Bit Operations/Bitwise Operator  logicop=AND  UseBitMask=on  BitMask=192  BitMaskRealWorld=Stored Integer
  EPB_Status_O : Constant  Value=0  OutDataTypeStr=single
  EPB_Status_S : ArithShift  BitShiftNumber=6
  EPB_Status_Sub : Subsystem
  EPB_Status_sat : Saturate  UpperLimit=3  LowerLimit=0
  EPB_Statuscv : DataTypeConversion
  EPB_FailStatus_Out : Outport
  EPB_Status_Out : Outport  Port=2
  EPB_FunctionLamp_Out : Outport  Port=3
  EPB_FailureLamp_Out : Outport  Port=4
  EPB_RollingCounter_id256_Out : Outport  Port=5
  EPB_Checksum_Out : Outport  Port=6
  wires:
  EPB_FailStatus_F/1 -> EPB_FailStatus_Ad/1
  EPB_FailStatus_O/1 -> EPB_FailStatus_Ad/2
  EPB_FailStatus_Ad/1 -> EPB_FailStatus_sat/1
  EPB_FailStatus_sat/1 -> EPB_FailStatus_Out/1
  Demux/1 -> EPB_FailStatus_Sub/1(In1)
  EPB_FailStatus_Sub/1(Out1) -> EPB_FailStatus_Convert/1
  EPB_FailStatus_Convert/1 -> EPB_FailStatus_L/1
  EPB_FailStatus_L/1 -> EPB_FailStatus_S/1
  EPB_FailStatus_S/1 -> EPB_FailStatuscv/1
  EPB_FailStatuscv/1 -> EPB_FailStatus_F/1
  EPB_Status_F/1 -> EPB_Status_Ad/1
  EPB_Status_O/1 -> EPB_Status_Ad/2
  EPB_Status_Ad/1 -> EPB_Status_sat/1
  EPB_Status_sat/1 -> EPB_Status_Out/1
  Demux/3 -> EPB_Status_Sub/1(In1)
  EPB_Status_Sub/1(Out1) -> EPB_Status_Convert/1
  EPB_Status_Convert/1 -> EPB_Status_L/1
  EPB_Status_L/1 -> EPB_Status_S/1
  EPB_Status_S/1 -> EPB_Statuscv/1
  EPB_Statuscv/1 -> EPB_Status_F/1
  EPB_FunctionLamp_F/1 -> EPB_FunctionLamp_Ad/1
  EPB_FunctionLamp_O/1 -> EPB_FunctionLamp_Ad/2
  EPB_FunctionLamp_Ad/1 -> EPB_FunctionLamp_sat/1
  EPB_FunctionLamp_sat/1 -> EPB_FunctionLamp_Out/1
  Demux/6 -> EPB_FunctionLamp_Sub/1(In1), EPB_FailureLamp_Sub/1(In1)
  EPB_FunctionLamp_Sub/1(Out1) -> EPB_FunctionLamp_Convert/1
  EPB_FunctionLamp_Convert/1 -> EPB_FunctionLamp_L/1
  EPB_FunctionLamp_L/1 -> EPB_FunctionLamp_S/1
  EPB_FunctionLamp_S/1 -> EPB_FunctionLampcv/1
  EPB_FunctionLampcv/1 -> EPB_FunctionLamp_F/1
  EPB_FailureLamp_F/1 -> EPB_FailureLamp_Ad/1
  EPB_FailureLamp_O/1 -> EPB_FailureLamp_Ad/2
  EPB_FailureLamp_Ad/1 -> EPB_FailureLamp_sat/1
  EPB_FailureLamp_sat/1 -> EPB_FailureLamp_Out/1
  EPB_FailureLamp_Sub/1(Out1) -> EPB_FailureLamp_Convert/1
  EPB_FailureLamp_Convert/1 -> EPB_FailureLamp_L/1
  EPB_FailureLamp_L/1 -> EPB_FailureLamp_S/1
  EPB_FailureLamp_S/1 -> EPB_FailureLampcv/1
  EPB_FailureLampcv/1 -> EPB_FailureLamp_F/1
  EPB_RollingCounter_id256_F/1 -> EPB_RollingCounter_id256_Ad/1
  EPB_RollingCounter_id256_O/1 -> EPB_RollingCounter_id256_Ad/2
  EPB_RollingCounter_id256_Ad/1 -> EPB_RollingCounter_id256_sat/1
  EPB_RollingCounter_id256_sat/1 -> EPB_RollingCounter_id256_Out/1
  Demux/7 -> EPB_RollingCounter_id256_Sub/1(In1)
  EPB_RollingCounter_id256_Sub/1(Out1) -> EPB_RollingCounter_id256_Convert/1
  EPB_RollingCounter_id256_Convert/1 -> EPB_RollingCounter_id256_L/1
  EPB_RollingCounter_id256_L/1 -> EPB_RollingCounter_id256_S/1
  EPB_RollingCounter_id256_S/1 -> EPB_RollingCounter_id256cv/1
  EPB_RollingCounter_id256cv/1 -> EPB_RollingCounter_id256_F/1
  EPB_Checksum_F/1 -> EPB_Checksum_Ad/1
  EPB_Checksum_O/1 -> EPB_Checksum_Ad/2
  EPB_Checksum_Ad/1 -> EPB_Checksum_sat/1
  EPB_Checksum_sat/1 -> EPB_Checksum_Out/1
  Demux/8 -> EPB_Checksum_Sub/1(In1)
  EPB_Checksum_Sub/1(Out1) -> EPB_Checksum_Convert/1
  EPB_Checksum_Convert/1 -> EPB_Checksum_L/1
  EPB_Checksum_L/1 -> EPB_Checksum_S/1
  EPB_Checksum_S/1 -> EPB_Checksumcv/1
  EPB_Checksumcv/1 -> EPB_Checksum_F/1
  input/1 -> Demux/1
